simulink model "adaptive_lms1"  (R2016b)
settings: Solver=VariableStepDiscrete  StartTime=0.0  StopTime=15  RelTol=1e-3  EnableMultiTasking=on
StartFcn:
  | tic
StopFcn:
  | toc
libraries: dspobslib x1, dspvision x1, dspadpt3 x1
settings Model: Creator=lcrockett  LastModifiedBy=Administrator
settings DataIOCC: LimitDataPoints=on  SaveFormat=Array  SignalLoggingSaveFormat=ModelDataLogs
settings OptimizationCC: DefaultParameterBehavior=Inlined  InlineInvariantSignals=on  ExpressionDepthLimit=2147483647  InitFltsAndDblsToZero=on  LifeSpan=inf
settings DebuggingCC: SaveWithParameterizedLinksMsg=none  UnderspecifiedInitializationDetection=Classic  MergeDetectMultiDrivingBlocksExec=none  SignalResolutionControl=TryResolveAllWithWarning  SolverPrmCheckMsg=warning  MultiTaskDSMMsg=warning  MultiTaskCondExecSysMsg=none  FcnCallInpInsideContextMsg=warning  StateNameClashWarn=warning  StrictBusMsg=None  SFUnexpectedBacktrackingDiag=warning  SFNoUnconditionalDefaultTransitionDiag=warning  SFExecutionAtInitializationDiag=none
settings HardwareCC: ProdBitPerPointer=32  ProdBitPerSizeT=32  ProdBitPerPtrDiffT=32  ProdLargestAtomicFloat=None  ProdIntDivRoundTo=Undefined  ProdEndianess=Unspecified  ProdWordSize=32  ProdHWDeviceType=32-bit Generic  TargetHWDeviceType=32-bit Generic  ProdEqTarget=off
settings ModelReferenceCC: PropagateSignalLabelsOutOfModel=off
settings GRTTargetCC: TargetFcnLib=ansi_tfl_tmw.mat  TargetLangStandard=C89/C90 (ANSI)  GeneratePreprocessorConditionals=Disable all  CombineOutputUpdateFcns=off  GRTInterface=on
settings ConfigComp: CovMetricSettings=dw  CovHtmlReporting=on  CovSaveCumulativeToWorkspaceVar=on  CovSaveSingleToWorkspaceVar=on  CovExternalEMLEnable=off

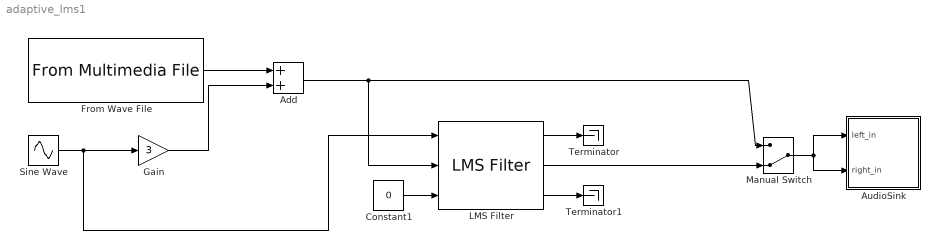
== system adaptive_lms1 ==
  Add : Sum
  AudioSink : Subsystem
  Constant1 : Constant  Value=0
  From Wave File : dspvision/From Multimedia File  inputFilename=E:\fpga_dsp_example\adaptive\lms_audio\Yabu_sample_48_mono.wav  loop=on  numPlays=1  outputStreams=Audio only  videoDataType=single  audioDataType=double  inheritSampleTime=on  userDefinedSampleTime=1/30  noAudioOutput=off  isIntensityVideo=off  fourcc=RGB  colorVideoFormat=Separate color signals  outputEOF=off  dataOrg=Column-major  audioFrameSize=1  computeAudioFrameSize=off  outSamplingMode=Sample based
  Gain : Gain  Gain=3
  LMS Filter : dspadpt3/LMS Filter  Algo=LMS  L=4  stepflag=Dialog  mu=0.001  leakage=1.0  ic=0  Adapt=off  resetflag=Non-zero sample  weights=on  secondCoeffMode=User-defined  secondCoeffWordLength=2  secondCoeffFracLength=15  accum2Mode=User-defined  accum2FracLength=20  prodOutput2Mode=User-defined  prodOutput2FracLength=20  prodOutput3Mode=User-defined  prodOutput3FracLength=20  prodOutput4Mode=User-defined  prodOutput4FracLength=20  quotientMode=User-defined  quotientFracLength=20  roundingMode=Floor  overflowMode=off  addnparflag=off
  Manual Switch : ManualSwitch  CurrentSetting=0
  Sine Wave : Sin  Amplitude=0.5  Frequency=2*pi*1200  SampleTime=1/48000  VectorParams1D=off
  Terminator : Terminator
  Terminator1 : Terminator
  wires:
  From Wave File/1 -> Add/1
  Sine Wave/1 -> LMS Filter/1, Gain/1
  Manual Switch/1 -> AudioSink/1(left_in), AudioSink/2(right_in)
  Add/1 -> LMS Filter/2, Manual Switch/1
  LMS Filter/2 -> Manual Switch/2
  Gain/1 -> Add/2
  LMS Filter/1 -> Terminator/1
  LMS Filter/3 -> Terminator1/1
  Constant1/1 -> LMS Filter/3

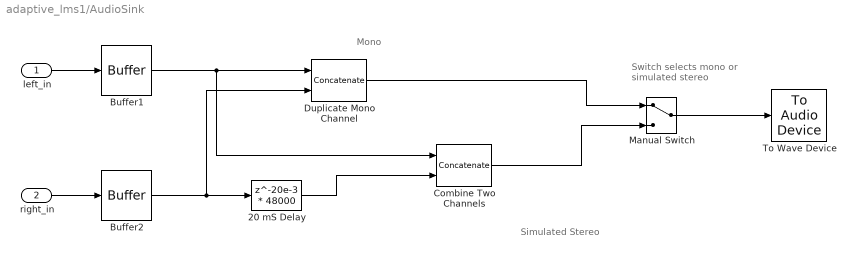
== system adaptive_lms1/AudioSink ==
  note: Mono
  note: Simulated
      | Stereo
  note: Switch selects mono
      | or simulated stereo
  left_in : Inport
  right_in : Inport  Port=2
  20 mS Delay : Delay  DelayLength=20e-3 * 48000  InitialCondition=0  InputProcessing=Inherited
  Buffer1 : Buffer  N=1
  Buffer2 : Buffer  N=1
  Combine Two Channels : Concatenate  Mode=Multidimensional array  ConcatenateDimension=2
  Duplicate Mono Channel : Concatenate  Mode=Multidimensional array  ConcatenateDimension=2
  Manual Switch : ManualSwitch
  To Wave Device : dspobslib/To Audio Device  deviceName=Default  inheritSampleRate=on  sampleRate=44100  deviceDatatype=Determine from input data type  autoBufferSize=on  bufferSize=4096  queueDuration=0.1  defaultOutputChannelMapping=on  outputChannelMapping=1:2  outputNumUnderrunSamples=off
  wires:
  20 mS Delay/1 -> Combine Two Channels/2
  Duplicate Mono Channel/1 -> Manual Switch/1
  left_in/1 -> Buffer1/1
  Manual Switch/1 -> To Wave Device/1
  Combine Two Channels/1 -> Manual Switch/2
  right_in/1 -> Buffer2/1
  Buffer2/1 -> Duplicate Mono Channel/2, 20 mS Delay/1
  Buffer1/1 -> Duplicate Mono Channel/1, Combine Two Channels/1
